simulink model "flightgear"  (R2026a)
settings: Solver=VariableStepAuto
libraries: aerolibfltsims x2
settings Model: Creator=vas77  LastModifiedBy=vas77

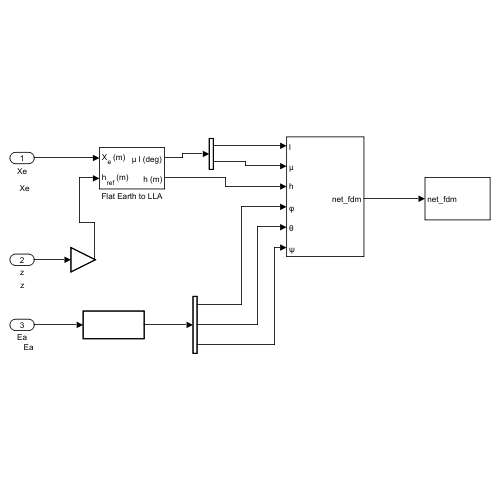
[thumbnail: Simulink's stored preview of the top-level diagram]
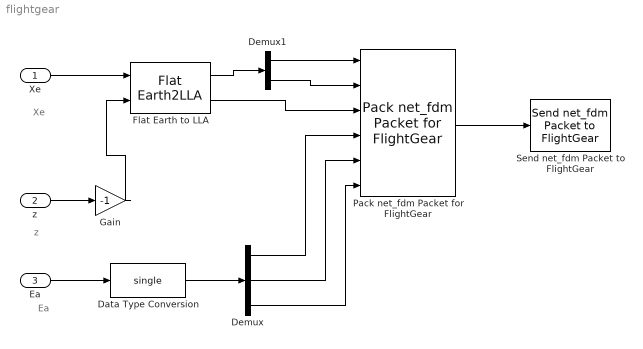
== system flightgear ==
  note: Ea
  note: z
  note: Xe
  Xe : Inport
  z : Inport  Port=2
  Ea : Inport  Port=3
  Data Type Conversion : DataTypeConversion  OutDataTypeStr=single  SaturateOnIntegerOverflow=off  RndMeth=Floor
  Demux : Demux  Outputs=3
  Demux1 : Demux  Outputs=2
  Flat Earth to LLA : FlatEarth2LLA
  Gain : Gain  Gain=-1
  Pack net_fdm Packet for FlightGear : aerolibfltsims/Pack net_fdm Packet for FlightGear  FlightGearVersion=v2019.1  ShowPositionAttitudeInputs=on  ShowVelocityAccelerationInputs=off  ShowControlSurfacePositionInputs=off  ShowEngineFuelInputs=off  ShowLandingGearInputs=off  ShowEnvironmentInputs=off  SampleTime=1/30  packetVersion=24
  Send net_fdm Packet to FlightGear : aerolibfltsims/Send net_fdm Packet to FlightGear  DestinationIpAddress=127.0.0.1  DestinationPort=5502  LocalIpPort=-1  varLen=off  SampleTime=1/30
  wires:
  z/1 -> Gain/1
  Pack net_fdm Packet for FlightGear/1 -> Send net_fdm Packet to FlightGear/1
  Ea/1 -> Data Type Conversion/1
  Data Type Conversion/1 -> Demux/1
  Demux/1 -> Pack net_fdm Packet for FlightGear/4
  Demux/2 -> Pack net_fdm Packet for FlightGear/5
  Demux/3 -> Pack net_fdm Packet for FlightGear/6
  Flat Earth to LLA/1 -> Demux1/1
  Demux1/1 -> Pack net_fdm Packet for FlightGear/1
  Demux1/2 -> Pack net_fdm Packet for FlightGear/2
  Flat Earth to LLA/2 -> Pack net_fdm Packet for FlightGear/3
  Gain/1 -> Flat Earth to LLA/2
  Xe/1 -> Flat Earth to LLA/1
